simulink model "CIE237_FINAL_STABLE123"  (R2025a)
settings: Solver=VariableStepAuto  StartTime=0.0  StopTime=1000  RelTol=1e-3
undefined symbols (not defined in the file): dspblkCoreblockFVToolHelper, gcbh
libraries: commsink2 x1, commrandsrc3 x1, dspsrcs4 x1, dspsigops x1
settings Model: Creator=compumarts  LastModifiedBy=compumarts

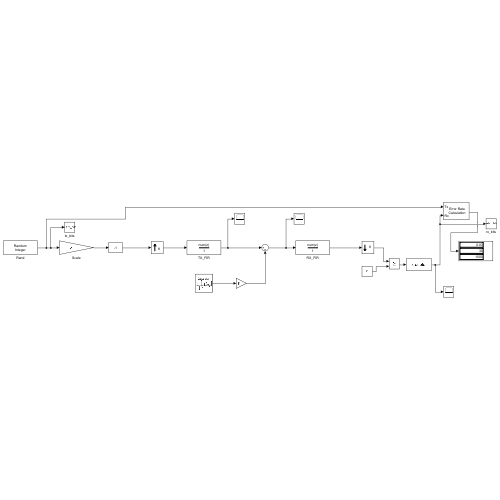
[thumbnail: Simulink's stored preview of the top-level diagram]
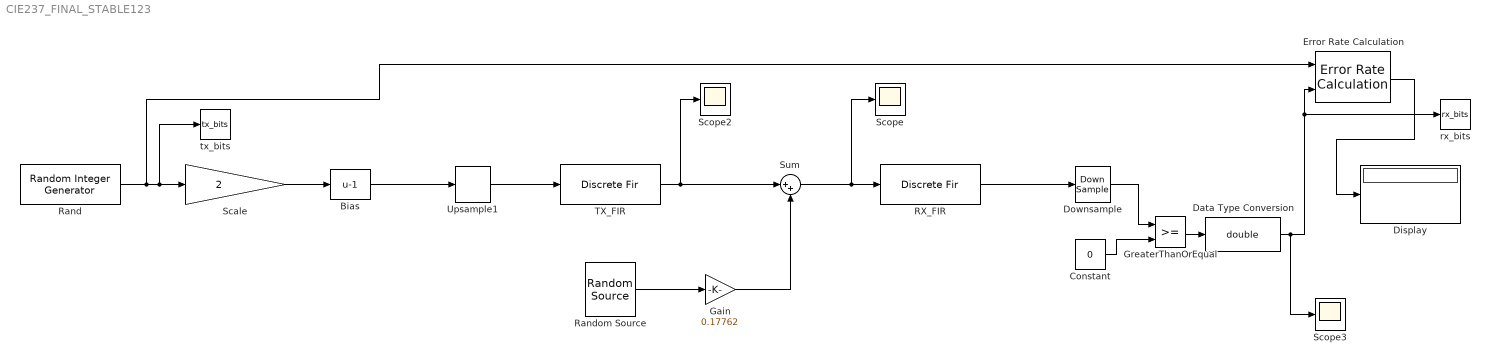
== system CIE237_FINAL_STABLE123 ==
  Bias : Bias  Bias=-1
  Constant : Constant  Value=0  OutDataTypeStr=double
  Data Type Conversion : DataTypeConversion  OutDataTypeStr=double  SaturateOnIntegerOverflow=off  RndMeth=Floor
  Display : Display
  Downsample : DownSample  N=8  RateOptions=Allow multirate processing  AllowArbitraryFixedInput=on
  Error Rate Calculation : commsink2/Error Rate Calculation  N=1  st_delay=0  cp_mode=Entire frame  subframe=[]  PMode=Port  WsName=BER_out  RsMode2=off  stop=off  numErr=100  maxBits=1e6
  Gain : Gain  Gain=0.17762
  GreaterThanOrEqual : RelationalOperator  OutDataTypeStr=boolean  RndMeth=Simplest  InputSameDT=off
  RX_FIR : DiscreteFir  LoadFcn=dspblkCoreblockFVToolHelper(gcbh,'load');  Coefficients=ones(1,8)/sqrt(8)  InputProcessing=Columns as channels (frame based)  OutDataTypeStr=Inherit: Same as input
      settings: CopyFcn=dspblkCoreblockFVToolHelper(gcbh,'copy');  DeleteFcn=dspblkCoreblockFVToolHelper(gcbh,'close');  ModelCloseFcn=dspblkCoreblockFVToolHelper(gcbh,'close');  PreSaveFcn=dspblkCoreblockFVToolHelper(gcbh,'presave');  PostSaveFcn=dspblkCoreblockFVToolHelper(gcbh,'postsave');  CloseFcn=dspblkCoreblockFVToolHelper(gcbh,'close');
  Rand : commrandsrc3/Random Integer Generator  SetSize=2  SeedSource=Auto  Seed=0  SampleTime=1  SamplesPerFrame=1  OutputDataType=double  SimulateUsing=Interpreted execution
  Random Source : dspsrcs4/Random Source  SrcType=Gaussian  MinVal=0  MaxVal=1  MeanVal=0  VarVal=1  RepMode=Specify seed  rawSeed=1  IsInherit=off  SampTime=1  SampFrame=1  OutComplex=Real  DataType=double  SimulateUsing=Interpreted execution
  Scale : Gain  Gain=2  OutDataTypeStr=Inherit: Inherit via back propagation  SaturateOnIntegerOverflow=on
  Scope : Scope
      settings: ActiveDisplayYMinimum=-1.272350461128084  ActiveDisplayYMaximum=1.7706105743706675
  Scope2 : Scope
      settings: ActiveDisplayYMinimum=-0.44194173824159216  ActiveDisplayYMaximum=0.44194173824159216  DataLoggingVariableName=ScopeData2
  Scope3 : Scope
      settings: ActiveDisplayYMinimum=-0.12499999999999997  ActiveDisplayYMaximum=1.125  DataLoggingVariableName=ScopeData3
  Sum : Sum  Inputs=|++
  TX_FIR : DiscreteFir  LoadFcn=dspblkCoreblockFVToolHelper(gcbh,'load');  Coefficients=ones(1,8)/sqrt(8)  InputProcessing=Columns as channels (frame based)  OutDataTypeStr=Inherit: Same as input
      settings: CopyFcn=dspblkCoreblockFVToolHelper(gcbh,'copy');  DeleteFcn=dspblkCoreblockFVToolHelper(gcbh,'close');  ModelCloseFcn=dspblkCoreblockFVToolHelper(gcbh,'close');  PreSaveFcn=dspblkCoreblockFVToolHelper(gcbh,'presave');  PostSaveFcn=dspblkCoreblockFVToolHelper(gcbh,'postsave');  CloseFcn=dspblkCoreblockFVToolHelper(gcbh,'close');
  Upsample1 : dspsigops/Upsample  FactorSource=Dialog parameter  N=8  Nmax=16  phase=0  RateOptions=Allow multirate processing  ic=0  mode=Unused parameter value
  rx_bits : ToWorkspace  VariableName=rx_bits  SampleTime=-1
  tx_bits : ToWorkspace  VariableName=tx_bits  SampleTime=-1
  wires:
  TX_FIR/1 -> Sum/1, Scope2/1
  Sum/1 -> Scope/1, RX_FIR/1
  Scale/1 -> Bias/1
  Bias/1 -> Upsample1/1
  Rand/1 -> Error Rate Calculation/1, tx_bits/1, Scale/1
  Upsample1/1 -> TX_FIR/1
  Downsample/1 -> GreaterThanOrEqual/1
  Constant/1 -> GreaterThanOrEqual/2
  GreaterThanOrEqual/1 -> Data Type Conversion/1
  Data Type Conversion/1 -> Scope3/1, rx_bits/1, Error Rate Calculation/2
  RX_FIR/1 -> Downsample/1
  Error Rate Calculation/1 -> Display/1
  Random Source/1 -> Gain/1
  Gain/1 -> Sum/2
